simulink model "Sepic_Zeta_CUK_Converter"  (R2023a)
settings: Solver=ode23t  StartTime=0.0  StopTime=10  MaxStep=1e-4  RelTol=1e-3
libraries: spsSeriesRLCBranchLib x17, spsCurrentMeasurementLib x3, spsDCVoltageSourceLib x3, spsDiodeLib x3, spsIGBTDiodeLib x3, spsVoltageMeasurementLib x3, sps_lib x1
settings Model: Creator=Alielden  LastModifiedBy=Alielden

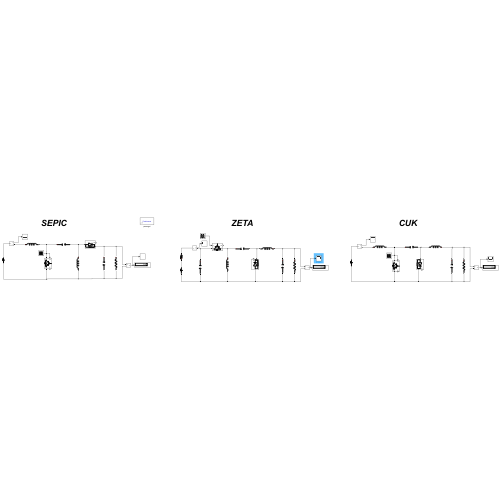
[thumbnail: Simulink's stored preview of the top-level diagram]
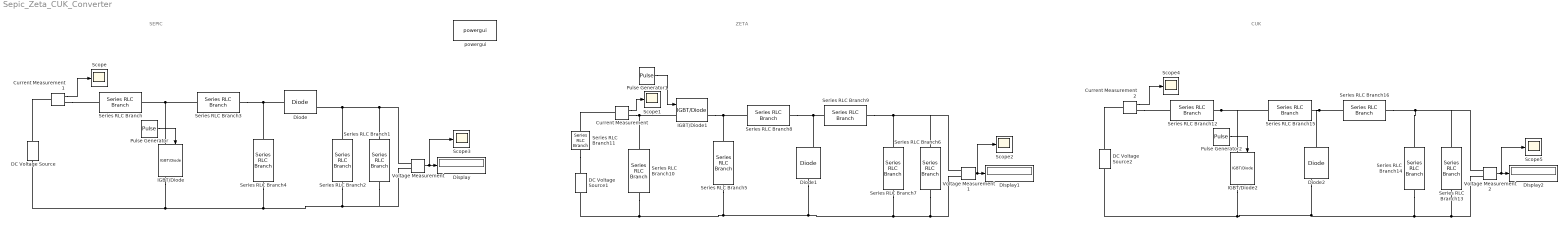
== system Sepic_Zeta_CUK_Converter ==
  note: ZETA
  note: SEPIC
  note: CUK
  Current Measurement : spsCurrentMeasurementLib/Current Measurement  PhasorSimulation=off  OutputType=Complex  PSBequivalent=0
  Current Measurement1 : spsCurrentMeasurementLib/Current Measurement  PhasorSimulation=off  OutputType=Complex  PSBequivalent=0
  Current Measurement2 : spsCurrentMeasurementLib/Current Measurement  PhasorSimulation=off  OutputType=Complex  PSBequivalent=0
  DC Voltage Source : spsDCVoltageSourceLib/DC Voltage Source  Amplitude=20  Measurements=None
  DC Voltage Source1 : spsDCVoltageSourceLib/DC Voltage Source  Amplitude=20  Measurements=None
  DC Voltage Source2 : spsDCVoltageSourceLib/DC Voltage Source  Amplitude=20  Measurements=None
  Diode : spsDiodeLib/Diode  Ron=0.001  Lon=0  Vf=0.8  IC=0  UseSnubber=0  Rs=500  Cs=250e-9  Measurements=on
  Diode1 : spsDiodeLib/Diode  Ron=0.001  Lon=0  Vf=0.8  IC=0  UseSnubber=0  Rs=500  Cs=250e-9  Measurements=on
  Diode2 : spsDiodeLib/Diode  Ron=0.001  Lon=0  Vf=0.8  IC=0  UseSnubber=0  Rs=500  Cs=250e-9  Measurements=on
  Display : Display
  Display1 : Display
  Display2 : Display
  IGBT/Diode : spsIGBTDiodeLib/IGBT//Diode  Ron=1e-3  Rs=1e5  Cs=inf  Measurements=on
  IGBT/Diode1 : spsIGBTDiodeLib/IGBT//Diode  Ron=1e-3  Rs=1e5  Cs=inf  Measurements=on
  IGBT/Diode2 : spsIGBTDiodeLib/IGBT//Diode  Ron=1e-3  Rs=1e5  Cs=inf  Measurements=on
  Pulse Generator : DiscretePulseGenerator  PulseType=Time based  Period=1/(10e3)  PulseWidth=80
  Pulse Generator1 : DiscretePulseGenerator  PulseType=Time based  Period=1/(10e3)  PulseWidth=80
  Pulse Generator2 : DiscretePulseGenerator  PulseType=Time based  Period=1/(10e3)  PulseWidth=80
  Scope{,1..5} (6 alike) : Scope
  Series RLC Branch{,4..5,9,12,16} (6 alike) : spsSeriesRLCBranchLib/Series RLC Branch  LConnTagsString=__new0  RConnTagsString=__new0  BranchType=L  Resistance=1  Inductance=8e-3  SetiL0=off  InitialCurrent=0  Capacitance=1e-6  Setx0=off  InitialVoltage=0  Measurements=None
  Series RLC Branch1 : spsSeriesRLCBranchLib/Series RLC Branch  LConnTagsString=__new0  RConnTagsString=__new0  BranchType=R  Resistance=80  Inductance=1e-3  SetiL0=off  InitialCurrent=0  Capacitance=1e-6  Setx0=off  InitialVoltage=0  Measurements=None
  Series RLC Branch10 : spsSeriesRLCBranchLib/Series RLC Branch  LConnTagsString=__new0  RConnTagsString=__new0  BranchType=C  Resistance=1  Inductance=1e-3  SetiL0=off  InitialCurrent=0  Capacitance=7400e-6  Setx0=off  InitialVoltage=0  Measurements=None
  Series RLC Branch11 : spsSeriesRLCBranchLib/Series RLC Branch  LConnTagsString=__new0  RConnTagsString=__new0  BranchType=R  Resistance=0.1  Inductance=1e-3  SetiL0=off  InitialCurrent=0  Capacitance=1e-6  Setx0=off  InitialVoltage=0  Measurements=None
  Series RLC Branch13 : spsSeriesRLCBranchLib/Series RLC Branch  LConnTagsString=__new0  RConnTagsString=__new0  BranchType=R  Resistance=80  Inductance=1e-3  SetiL0=off  InitialCurrent=0  Capacitance=1e-6  Setx0=off  InitialVoltage=0  Measurements=None
  Series RLC Branch{2..3,7..8,14..15} (6 alike) : spsSeriesRLCBranchLib/Series RLC Branch  LConnTagsString=__new0  RConnTagsString=__new0  BranchType=C  Resistance=1  Inductance=1e-3  SetiL0=off  InitialCurrent=0  Capacitance=800e-6  Setx0=off  InitialVoltage=0  Measurements=None
  Series RLC Branch6 : spsSeriesRLCBranchLib/Series RLC Branch  LConnTagsString=__new0  RConnTagsString=__new0  BranchType=R  Resistance=80  Inductance=1e-3  SetiL0=off  InitialCurrent=0  Capacitance=1e-6  Setx0=off  InitialVoltage=0  Measurements=None
  Voltage Measurement : spsVoltageMeasurementLib/Voltage Measurement  PhasorSimulation=off  OutputType=Complex  PSBequivalent=0
  Voltage Measurement1 : spsVoltageMeasurementLib/Voltage Measurement  PhasorSimulation=off  OutputType=Complex  PSBequivalent=0
  Voltage Measurement2 : spsVoltageMeasurementLib/Voltage Measurement  PhasorSimulation=off  OutputType=Complex  PSBequivalent=0
  powergui : sps_lib/powergui  Priority=1  SimulationMode=Continuous  SampleTime=1e-6  frequency=60  Iterations=50  frequencyindice=0  Pbase=100e6  ErrMax=1e-4  UnitsV=kV  UnitsW=MW  buscounter=0  FunctionMessages=off  echomessages=off  EnableUseOfTLC=off  CurrentSourceSwitches=off  DisableSnubberDevices=off  DisableRonSwitches=off  DisableVfSwitches=off  DisplayEquations=off  AutomaticDiscreteSolvers=off  SolverType=Tustin/Backward Euler (TBE)  Interpol=off  ExternalGateDelay=off  methode=off  Ts=100  x0status=blocks  SPID=on  SwTol=0  HookPort=off  NonlinearTolerance=1e-4  nMaxIteration=100  ContinueOnMaxIteration=off  RestoreLinks=warning  ResistiveCurrentMeasurement=off  Frange=[0:2:500]  Ylog=off  Xlog=on  ShowGrid=off  save=off  variable=ZData  structure=0  ZoomFFT=off  StartTime=0.0  cycles=1  DisplayStyle=1  fundamental=60  FreqAxis=off  MaxFrequency=1000  frequencyindicesteady=1  RmsSteady=1  display=off
  wires:
  Pulse Generator/1 -> IGBT/Diode/1
  Pulse Generator1/1 -> IGBT/Diode1/1
  Current Measurement1/1 -> Scope/1
  Current Measurement/1 -> Scope1/1
  Voltage Measurement1/1 -> Scope2/1, Display1/1
  Voltage Measurement/1 -> Scope3/1, Display/1
  Voltage Measurement2/1 -> Scope5/1, Display2/1
  Current Measurement2/1 -> Scope4/1
  Pulse Generator2/1 -> IGBT/Diode2/1
  connections:
  Series RLC Branch2/RConn1 -- Series RLC Branch4/RConn1 -- IGBT/Diode/RConn1 -- DC Voltage Source/LConn1 -- Voltage Measurement/LConn2 -- Series RLC Branch1/RConn1
  Series RLC Branch1/LConn1 -- Voltage Measurement/LConn1 -- Series RLC Branch2/LConn1 -- Diode/RConn1
  Series RLC Branch3/RConn1 -- Diode/LConn1 -- Series RLC Branch4/LConn1
  IGBT/Diode/LConn1 -- Series RLC Branch3/LConn1 -- Series RLC Branch/RConn1
  Series RLC Branch6/LConn1 -- Voltage Measurement1/LConn1 -- Series RLC Branch9/LConn1 -- Series RLC Branch7/LConn1
  Series RLC Branch6/RConn1 -- Voltage Measurement1/LConn2 -- Series RLC Branch7/RConn1 -- Diode1/LConn1 -- Series RLC Branch5/RConn1 -- Series RLC Branch10/RConn1 -- DC Voltage Source1/LConn1
  Series RLC Branch8/RConn1 -- Series RLC Branch9/RConn1 -- Diode1/RConn1
  Series RLC Branch5/LConn1 -- Series RLC Branch8/LConn1 -- IGBT/Diode1/RConn1
  Current Measurement/RConn1 -- Series RLC Branch10/LConn1 -- IGBT/Diode1/LConn1
  Current Measurement1/RConn1 -- Series RLC Branch/LConn1
  Current Measurement1/LConn1 -- DC Voltage Source/RConn1
  Series RLC Branch11/LConn1 -- DC Voltage Source1/RConn1
  Series RLC Branch11/RConn1 -- Current Measurement/LConn1
  Series RLC Branch12/RConn1 -- IGBT/Diode2/LConn1 -- Series RLC Branch15/LConn1
  Series RLC Branch13/LConn1 -- Voltage Measurement2/LConn1 -- Series RLC Branch14/LConn1 -- Series RLC Branch16/LConn1
  Series RLC Branch13/RConn1 -- Voltage Measurement2/LConn2 -- Series RLC Branch14/RConn1 -- Diode2/RConn1 -- IGBT/Diode2/RConn1 -- DC Voltage Source2/LConn1
  Current Measurement2/LConn1 -- DC Voltage Source2/RConn1
  Current Measurement2/RConn1 -- Series RLC Branch12/LConn1
  Diode2/LConn1 -- Series RLC Branch16/RConn1 -- Series RLC Branch15/RConn1
